simulink model "Traditional_MPC_MMC_qudratic"  (R2019b)
settings: Solver=ode3  StartTime=0.0  StopTime=3  FixedStep=0.000050  RelTol=1e-3  EnableMultiTasking=on
settings Model: Creator=cary  LastModifiedBy=adshetgaonkar
settings DataIOCC: LimitDataPoints=on  SaveFormat=Array  SignalLoggingSaveFormat=ModelDataLogs  ReturnWorkspaceOutputs=off
settings OptimizationCC: ExpressionDepthLimit=2147483647  LifeSpan=1  EfficientTunableParamExpr=on
settings DebuggingCC: UnderspecifiedInitializationDetection=Classic  MergeDetectMultiDrivingBlocksExec=none  SolverPrmCheckMsg=warning  FcnCallInpInsideContextMsg=warning  StateNameClashWarn=warning  SFUnexpectedBacktrackingDiag=warning  SFNoUnconditionalDefaultTransitionDiag=warning  SFExecutionAtInitializationDiag=none  ArithmeticOperatorsInVariantConditions=warning
settings HardwareCC: ProdBitPerPointer=32  ProdBitPerSizeT=32  ProdBitPerPtrDiffT=32  ProdLargestAtomicFloat=None  ProdIntDivRoundTo=Undefined  ProdEndianess=Unspecified  ProdWordSize=32  ProdHWDeviceType=32-bit Generic
settings ModelReferenceCC: PropagateSignalLabelsOutOfModel=off
settings SFSimCC: SimUseLocalCustomCode=off  MATLABDynamicMemAlloc=off  CustomCodeUndefinedFunction=UseInterfaceOnly
settings RTWCC: SystemTargetFile=ert.tlc  TemplateMakefile=ert_default_tmf  RTWUseLocalCustomCode=off
settings CodeAppCC: IgnoreCustomStorageClasses=off  CustomSymbolStrType=$N$R$M  StateflowObjectComments=on  InternalIdentifier=Classic
settings ERTTargetCC: MultiwordLength=2048  GenerateSampleERTMain=on  IncludeMdlTerminateFcn=off  SupportComplex=off  SupportContinuousTime=on  ERTCustomFileTemplate=example_file_process.tlc  ConvertIfToSwitch=off  SuppressUnreachableDefaultCases=off
settings ConfigComp: CovMetricSettings=dw  CovHtmlReporting=on  CovSaveCumulativeToWorkspaceVar=on  CovSaveSingleToWorkspaceVar=on  CovExternalEMLEnable=off

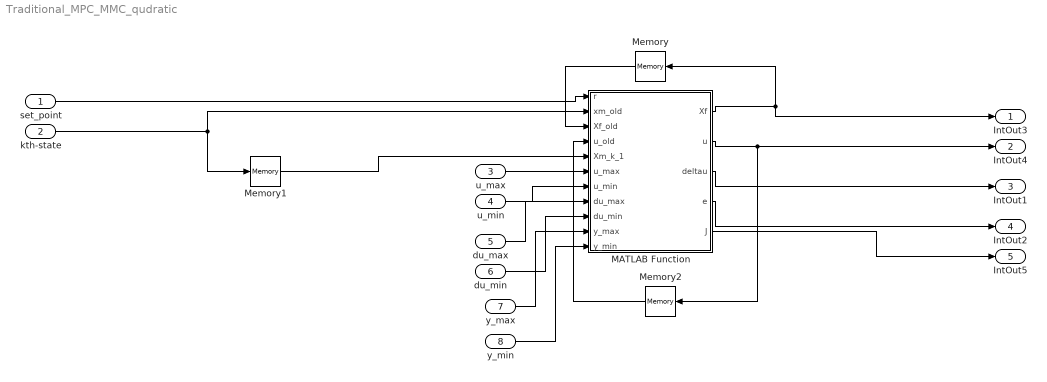
== system Traditional_MPC_MMC_qudratic ==
  set_point : Inport  PortDimensions=5
  kth-state : Inport  Port=2  PortDimensions=5
  u_max : Inport  Port=3  PortDimensions=5
  u_min : Inport  Port=4  PortDimensions=5
  du_max : Inport  Port=5  PortDimensions=1
  du_min : Inport  Port=6  PortDimensions=1
  y_max : Inport  Port=7  PortDimensions=1
  y_min : Inport  Port=8  PortDimensions=1
  MATLAB Function : MATLAB Function  TreatAsAtomicUnit=on
  Memory : Memory
  Memory1 : Memory
  Memory2 : Memory
  IntOut3 : Outport  SignalName=Xf
  IntOut4 : Outport  Port=2  SignalName=u
  IntOut1 : Outport  Port=3  SignalName=delta_u
  IntOut2 : Outport  Port=4  SignalName=error
  IntOut5 : Outport  Port=5  SignalName=J
  wires:
  set_point/1 -> MATLAB Function/1(r)
  MATLAB Function/1(Xf) -> IntOut3/1, Memory/1
  kth-state/1 -> MATLAB Function/2(xm_old), Memory1/1
  MATLAB Function/3(deltau) -> IntOut1/1
  Memory1/1 -> MATLAB Function/5(Xm_k_1)
  Memory/1 -> MATLAB Function/3(Xf_old)
  Memory2/1 -> MATLAB Function/4(u_old)
  MATLAB Function/2(u) -> Memory2/1, IntOut4/1
  u_max/1 -> MATLAB Function/6(u_max)
  u_min/1 -> MATLAB Function/7(u_min)
  MATLAB Function/4(e) -> IntOut2/1
  du_min/1 -> MATLAB Function/9(du_min)
  du_max/1 -> MATLAB Function/8(du_max)
  y_max/1 -> MATLAB Function/10(y_max)
  y_min/1 -> MATLAB Function/11(y_min)
  MATLAB Function/5(J) -> IntOut5/1

== matlab function Traditional_MPC_MMC_qudratic/MATLAB Function ==
  data: r input; Xf output; xm_old input; u output; Xf_old input; u_old input; Xm_k_1 input; deltau output; u_max input; u_min input; e output; du_max input; du_min input; y_max input; y_min input; J output
function [Xf,u,deltau,e,J] = fcn(r,xm_old,Xf_old,u_old,Xm_k_1,u_max,u_min,du_max,du_min,y_max,y_min)
D = []; 
D= coder.load('initial_qudratic_paper_traditional_MPC.mat'); 

%%% model-plant mismatch error 
xm=D.Ap*xm_old+D.Bp*(u_old+D.up);
y_model=D.Cp*xm;
e = (y_model - xm_old); 
g = -(D.PhiT_Q_R_bar*r- D.PhiT_Q_F*(D.Xf+Xf_old)- D.PhiT_Q_Ie*(D.e+e)); 
%%% with one step output constraint there is no time over flow
B_LHS=[D.bduMax*du_max;-D.bduMin*du_min; D.Iu*(u_max-u_old);-D.Iu*(u_min-u_old);y_max-D.F(159,:)*(D.Xf+Xf_old);-y_min+D.F(159,:)*(D.Xf+Xf_old)]; %%F(4,:) indicate k+1 
%B_LHS=[D.bduMax*du_max;-D.bduMin*du_min; D.Iu*(u_max-u_old);-D.Iu*(u_min-u_old)];
%DeltaU = -D.H\g;
DeltaU = QPhild(D.H,g,D.C_LHS,B_LHS);
deltau= DeltaU(1:D.m,:);
J = DeltaU'*D.H*DeltaU + 2*DeltaU'*g;
u=D.up+u_old+deltau;
y = xm_old;
y_delta_k=y-Xm_k_1;
Xf=[y_delta_k;y];
end
